simulink model "Longitudinal_Simulink_MaskedParameter_WithOutput"  (Simulink 7.1)
settings: Solver=ode45  StartTime=0.0  StopTime=2.0  RelTol=1e-3
settings Model: Creator=Meisel  LastModifiedBy=Meisel

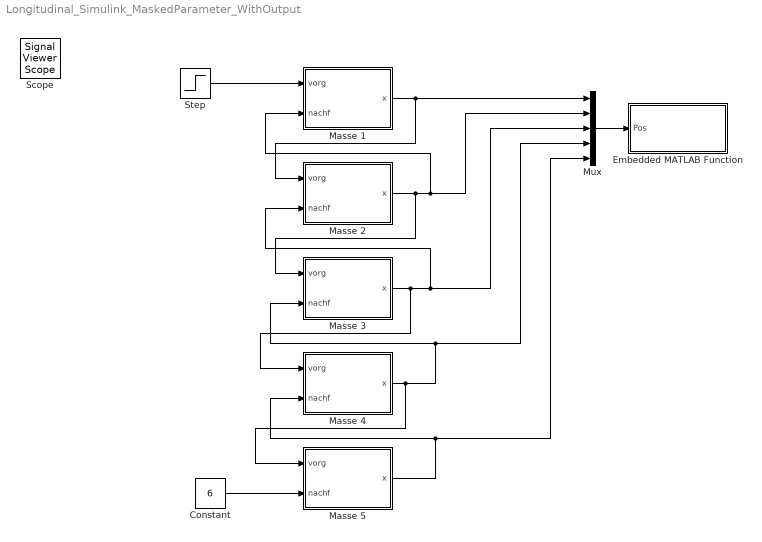
== system Longitudinal_Simulink_MaskedParameter_WithOutput ==
  Constant : Constant  Value=6  OutDataType=sfix(16)  OutScaling=2^0
  Embedded MATLAB Function : Stateflow chart
  Masse 1 : Subsystem  mask{Init_Pos=1}
      mask prompts: Init_Pos "Startposition"
  Masse 2 : Subsystem  mask{Init_Pos=2}
      mask prompts: Init_Pos "Startposition"
  Masse 3 : Subsystem  mask{Init_Pos=3}
      mask prompts: Init_Pos "Startposition"
  Masse 4 : Subsystem  mask{Init_Pos=4}
      mask prompts: Init_Pos "Startposition"
  Masse 5 : Subsystem  mask{Init_Pos=5}
      mask prompts: Init_Pos "Startposition"
  Mux : Mux  Inputs=5
  Step : Step  Time=0  After=0.5  SampleTime=0
  Scope : SignalViewerScope  IOType=viewer  RefreshTime=0.035000
      settings: YMin=0  YMax=0.1
  wires:
  Masse 1/1(x) -> Mux/1, Masse 2/1(vorg)
  Step/1 -> Masse 1/1(vorg)
  Masse 2/1(x) -> Masse 3/1(vorg), Masse 1/2(nachf), Mux/2
  Masse 3/1(x) -> Masse 4/1(vorg), Masse 2/2(nachf), Mux/3
  Masse 4/1(x) -> Masse 5/1(vorg), Masse 3/2(nachf), Mux/4
  Masse 5/1(x) -> Masse 4/2(nachf), Mux/5
  Constant/1 -> Masse 5/2(nachf)
  Mux/1 -> Embedded MATLAB Function/1(Pos)

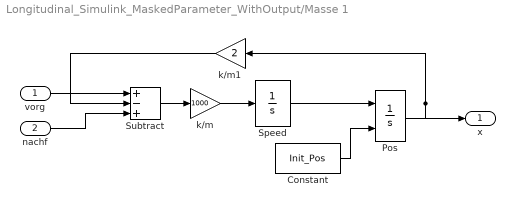
== system Longitudinal_Simulink_MaskedParameter_WithOutput/Masse 1 ==
  vorg : Inport  OutDataType=sfix(16)  OutScaling=2^0
  nachf : Inport  Port=2  OutDataType=sfix(16)  OutScaling=2^0
  Constant : Constant  Value=Init_Pos  OutDataType=sfix(16)  OutScaling=2^0
  Pos : Integrator  InitialConditionSource=external  InitialCondition=1
  Speed : Integrator
  Subtract : Sum  Inputs=+-+  OutDataType=sfix(16)  OutScaling=2^-10
  k/m : Gain  Gain=1000  ParameterDataType=sfix(16)  ParameterScaling=2^0  OutDataType=sfix(16)  OutScaling=2^0
  k/m1 : Gain  Orientation=left  Gain=2  ParameterDataType=sfix(16)  ParameterScaling=2^0  OutDataType=sfix(16)  OutScaling=2^0
  x : Outport  OutDataType=sfix(16)  OutScaling=2^0
  wires:
  Speed/1 -> Pos/1
  Subtract/1 -> k/m/1
  k/m/1 -> Speed/1
  Pos/1 -> x/1, k/m1/1
  nachf/1 -> Subtract/3
  vorg/1 -> Subtract/1
  k/m1/1 -> Subtract/2
  Constant/1 -> Pos/2

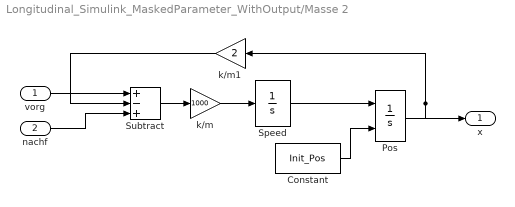
== system Longitudinal_Simulink_MaskedParameter_WithOutput/Masse 2 ==
  vorg : Inport  OutDataType=sfix(16)  OutScaling=2^0
  nachf : Inport  Port=2  OutDataType=sfix(16)  OutScaling=2^0
  Constant : Constant  Value=Init_Pos  OutDataType=sfix(16)  OutScaling=2^0
  Pos : Integrator  InitialConditionSource=external  InitialCondition=1
  Speed : Integrator
  Subtract : Sum  Inputs=+-+  OutDataType=sfix(16)  OutScaling=2^-10
  k/m : Gain  Gain=1000  ParameterDataType=sfix(16)  ParameterScaling=2^0  OutDataType=sfix(16)  OutScaling=2^0
  k/m1 : Gain  Orientation=left  Gain=2  ParameterDataType=sfix(16)  ParameterScaling=2^0  OutDataType=sfix(16)  OutScaling=2^0
  x : Outport  OutDataType=sfix(16)  OutScaling=2^0
  wires:
  Speed/1 -> Pos/1
  Subtract/1 -> k/m/1
  k/m/1 -> Speed/1
  Pos/1 -> x/1, k/m1/1
  nachf/1 -> Subtract/3
  vorg/1 -> Subtract/1
  k/m1/1 -> Subtract/2
  Constant/1 -> Pos/2

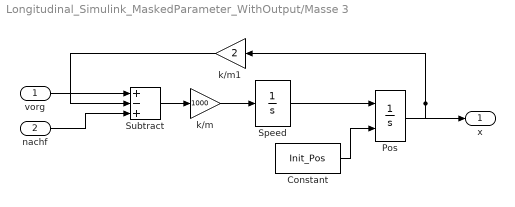
== system Longitudinal_Simulink_MaskedParameter_WithOutput/Masse 3 ==
  vorg : Inport  OutDataType=sfix(16)  OutScaling=2^0
  nachf : Inport  Port=2  OutDataType=sfix(16)  OutScaling=2^0
  Constant : Constant  Value=Init_Pos  OutDataType=sfix(16)  OutScaling=2^0
  Pos : Integrator  InitialConditionSource=external  InitialCondition=1
  Speed : Integrator
  Subtract : Sum  Inputs=+-+  OutDataType=sfix(16)  OutScaling=2^-10
  k/m : Gain  Gain=1000  ParameterDataType=sfix(16)  ParameterScaling=2^0  OutDataType=sfix(16)  OutScaling=2^0
  k/m1 : Gain  Orientation=left  Gain=2  ParameterDataType=sfix(16)  ParameterScaling=2^0  OutDataType=sfix(16)  OutScaling=2^0
  x : Outport  OutDataType=sfix(16)  OutScaling=2^0
  wires:
  Speed/1 -> Pos/1
  Subtract/1 -> k/m/1
  k/m/1 -> Speed/1
  Pos/1 -> x/1, k/m1/1
  nachf/1 -> Subtract/3
  vorg/1 -> Subtract/1
  k/m1/1 -> Subtract/2
  Constant/1 -> Pos/2

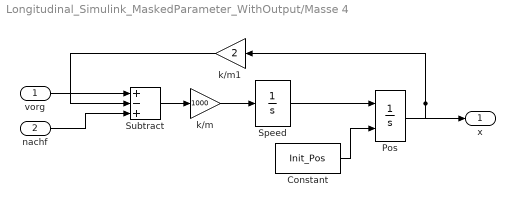
== system Longitudinal_Simulink_MaskedParameter_WithOutput/Masse 4 ==
  vorg : Inport  OutDataType=sfix(16)  OutScaling=2^0
  nachf : Inport  Port=2  OutDataType=sfix(16)  OutScaling=2^0
  Constant : Constant  Value=Init_Pos  OutDataType=sfix(16)  OutScaling=2^0
  Pos : Integrator  InitialConditionSource=external  InitialCondition=1
  Speed : Integrator
  Subtract : Sum  Inputs=+-+  OutDataType=sfix(16)  OutScaling=2^-10
  k/m : Gain  Gain=1000  ParameterDataType=sfix(16)  ParameterScaling=2^0  OutDataType=sfix(16)  OutScaling=2^0
  k/m1 : Gain  Orientation=left  Gain=2  ParameterDataType=sfix(16)  ParameterScaling=2^0  OutDataType=sfix(16)  OutScaling=2^0
  x : Outport  OutDataType=sfix(16)  OutScaling=2^0
  wires:
  Speed/1 -> Pos/1
  Subtract/1 -> k/m/1
  k/m/1 -> Speed/1
  Pos/1 -> x/1, k/m1/1
  nachf/1 -> Subtract/3
  vorg/1 -> Subtract/1
  k/m1/1 -> Subtract/2
  Constant/1 -> Pos/2

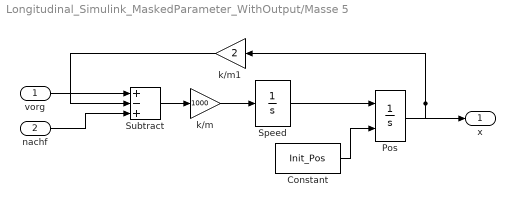
== system Longitudinal_Simulink_MaskedParameter_WithOutput/Masse 5 ==
  vorg : Inport  OutDataType=sfix(16)  OutScaling=2^0
  nachf : Inport  Port=2  OutDataType=sfix(16)  OutScaling=2^0
  Constant : Constant  Value=Init_Pos  OutDataType=sfix(16)  OutScaling=2^0
  Pos : Integrator  InitialConditionSource=external  InitialCondition=1
  Speed : Integrator
  Subtract : Sum  Inputs=+-+  OutDataType=sfix(16)  OutScaling=2^-10
  k/m : Gain  Gain=1000  ParameterDataType=sfix(16)  ParameterScaling=2^0  OutDataType=sfix(16)  OutScaling=2^0
  k/m1 : Gain  Orientation=left  Gain=2  ParameterDataType=sfix(16)  ParameterScaling=2^0  OutDataType=sfix(16)  OutScaling=2^0
  x : Outport  OutDataType=sfix(16)  OutScaling=2^0
  wires:
  Speed/1 -> Pos/1
  Subtract/1 -> k/m/1
  k/m/1 -> Speed/1
  Pos/1 -> x/1, k/m1/1
  nachf/1 -> Subtract/3
  vorg/1 -> Subtract/1
  k/m1/1 -> Subtract/2
  Constant/1 -> Pos/2

== matlab function Embedded MATLAB Function ==
  data: Pos input double
function OutScatter(Pos)
% Embedded MATLAB  

eml.extrinsic('set', 'drawnow', 'scatter', 'gca');
persistent y l0;

    % Init-Parameter
    k  = 5;             % Anzahl der Massen
    l0 = 1;             % Abstand zwischen den Massen
       
    % y-Werte anlegen und mit 0 initialisieren
    y=zeros(1,k);    
   
    % Scatterplot zeichnen
    scatter(Pos', y,  'o', 'MarkerFaceColor', [1 0 0]);
    set (gca,'XLim', [0 (k+1)*l0] );  % x-Bereich festhalten
    drawnow;                          % jetzt zeichnen
end
